simulink model "cruise_control_fechada"  (R2022b)
settings: Solver=FixedStepAuto  StartTime=0.0  StopTime=100  FixedStep=1e-3  RelTol=1e-3
values from neighbouring files (symbols this model uses):
  b = f/v(end)    [identificarCruiseControl.m]
  m = -b * t(1000) / log(1 - (b/f) * v(1000))    [identificarCruiseControl.m]
undefined symbols (not defined in the file or in its folder): bc, d, Kp, vr
settings Model: Creator=mmaximo  LastModifiedBy=danie
settings SolverCC: AlgebraicLoopSolver=TrustRegion
settings DebuggingCC: UnconnectedInputMsg=warning  UnconnectedOutputMsg=warning  UnconnectedLineMsg=warning  SFMachineParentedDataDiag=warning
settings ModelReferenceCC: EnableRefExpFcnMdlSchedulingChecks=on
settings RTWCC: DLArmComputeVersion=19.05

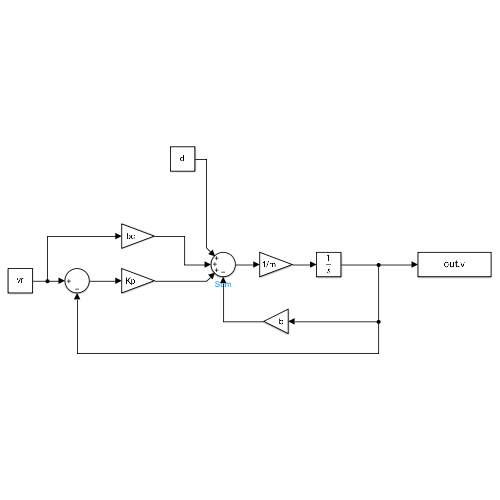
[thumbnail: Simulink's stored preview of the top-level diagram]
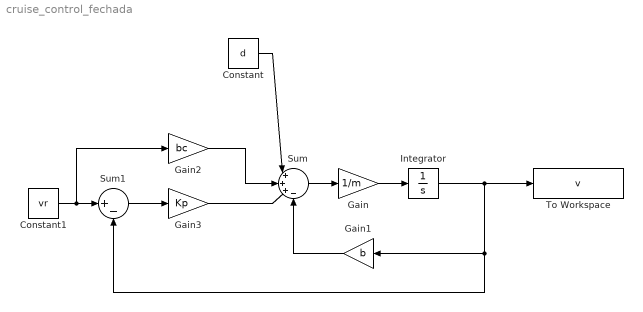
== system cruise_control_fechada ==
  Constant : Constant  Value=d
  Constant1 : Constant  Value=vr
  Gain : Gain  Gain=1/m
  Gain1 : Gain  Gain=b
  Gain2 : Gain  Gain=bc
  Gain3 : Gain  Gain=Kp
  Integrator : Integrator
  Sum : Sum  Inputs=|+++-
  Sum1 : Sum  Inputs=|+-
  To Workspace : ToWorkspace  VariableName=v  SaveFormat=Structure With Time  SampleTime=-1
  wires:
  Gain2/1 -> Sum/2
  Constant/1 -> Sum/1
  Sum/1 -> Gain/1
  Gain/1 -> Integrator/1
  Integrator/1 -> Gain1/1, Sum1/2, To Workspace/1
  Gain3/1 -> Sum/3
  Constant1/1 -> Gain2/1, Sum1/1
  Sum1/1 -> Gain3/1
  Gain1/1 -> Sum/4
